simulink model "przestrzen_stanu_1"  (R2014b)
settings: Solver=FixedStepDiscrete  StartTime=0.0  StopTime=100.0  RelTol=1e-3
values from neighbouring files (symbols this model uses):
  x0 = [ 10 1 10 ]    [zad_4.m]
undefined symbols (not defined in the file or in its folder): A1, C1, Tp
settings Model: Creator=Konrad  LastModifiedBy=Konrad

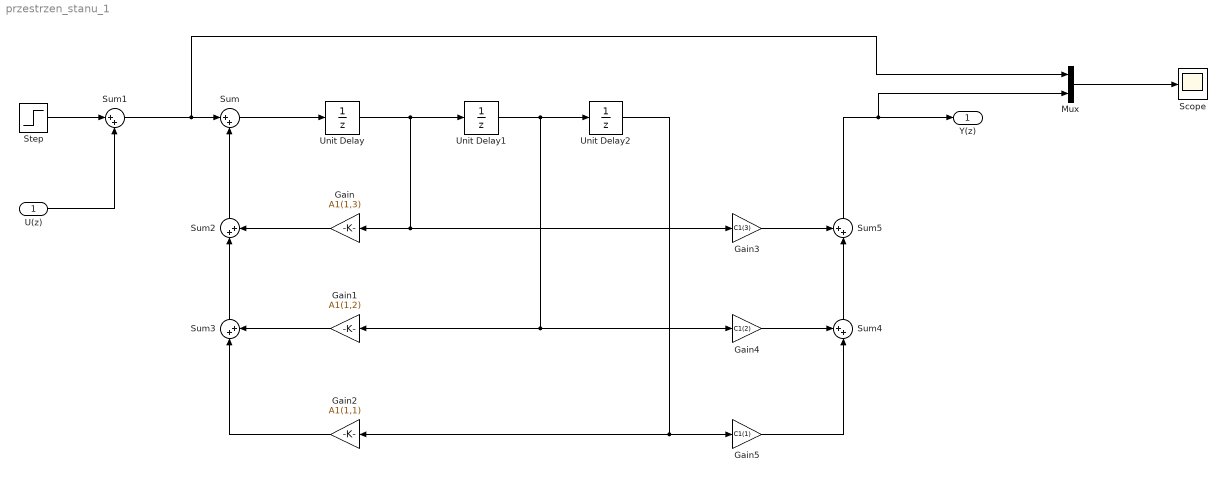
== system przestrzen_stanu_1 ==
  U(z) : Inport
  Gain : Gain  Gain=A1(1,3)
  Gain1 : Gain  Gain=A1(1,2)
  Gain2 : Gain  Gain=A1(1,1)
  Gain3 : Gain  Gain=C1(3)
  Gain4 : Gain  Gain=C1(2)
  Gain5 : Gain  Gain=C1(1)
  Mux : Mux  Inputs=2
  Scope : Scope
  Step : Step  SampleTime=0
  Sum{,1..3} (4 alike) : Sum  Inputs=|++
  Sum4 : Sum  Inputs=++|
  Sum5 : Sum  Inputs=++|
  Unit Delay : UnitDelay  InitialCondition=x0(1)  SampleTime=Tp
  Unit Delay1 : UnitDelay  InitialCondition=x0(2)  SampleTime=Tp
  Unit Delay2 : UnitDelay  InitialCondition=x0(3)  SampleTime=Tp
  Y(z) : Outport
  wires:
  Unit Delay/1 -> Unit Delay1/1, Gain3/1, Gain/1
  Unit Delay1/1 -> Unit Delay2/1, Gain4/1, Gain1/1
  Sum/1 -> Unit Delay/1
  Sum2/1 -> Sum/2
  Sum3/1 -> Sum2/1
  Gain2/1 -> Sum3/1
  Unit Delay2/1 -> Gain5/1, Gain2/1
  Gain1/1 -> Sum3/2
  Gain/1 -> Sum2/2
  Gain4/1 -> Sum4/1
  Gain3/1 -> Sum5/1
  Gain5/1 -> Sum4/2
  Sum4/1 -> Sum5/2
  Sum1/1 -> Mux/1, Sum/1
  Sum5/1 -> Mux/2, Y(z)/1
  Step/1 -> Sum1/1
  U(z)/1 -> Sum1/2
  Mux/1 -> Scope/1
